simulink model "ThreePhase_FullControlRectifier"  (R2020a)
settings: Solver=VariableStepAuto  StartTime=0.0  StopTime=0.0335  RelTol=1e-3
libraries: powerlib x15
settings Model: Creator=Naeem Mohammad  LastModifiedBy=Naeem Mohammad

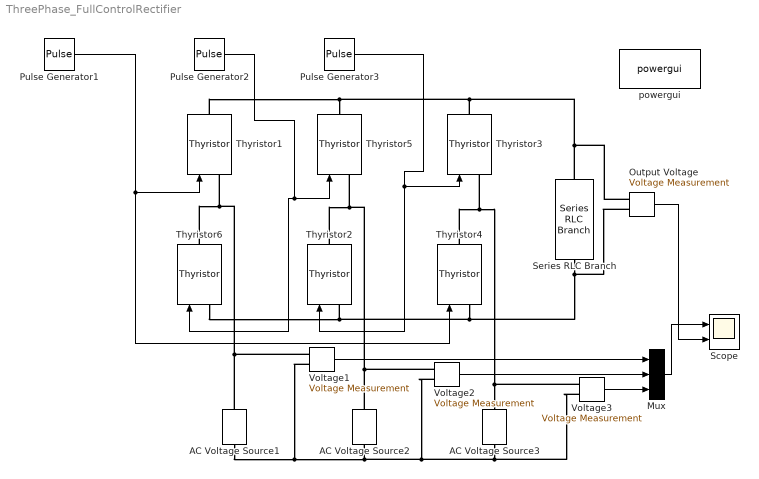
== system ThreePhase_FullControlRectifier ==
  AC Voltage Source1 : powerlib/Electrical Sources/AC Voltage Source  Amplitude=220  Phase=0  Frequency=60  SampleTime=0  Measurements=None  BusType=swing  Pref=10e3  Qref=0  Qmin=-inf  Qmax=+inf
  AC Voltage Source2 : powerlib/Electrical Sources/AC Voltage Source  Amplitude=220  Phase=120  Frequency=60  SampleTime=0  Measurements=None  BusType=swing  Pref=10e3  Qref=0  Qmin=-inf  Qmax=+inf
  AC Voltage Source3 : powerlib/Electrical Sources/AC Voltage Source  Amplitude=220  Phase=240  Frequency=60  SampleTime=0  Measurements=None  BusType=swing  Pref=10e3  Qref=0  Qmin=-inf  Qmax=+inf
  Mux : Mux  Inputs=3
  Output Voltage : powerlib/Measurements/Voltage Measurement  PhasorSimulation=off  OutputType=Complex  PSBequivalent=0
  Pulse Generator1 : DiscretePulseGenerator  PulseType=Time based  Period=1/60  PulseWidth=5  PhaseDelay=45*(1/60)*(1/360)
  Pulse Generator2 : DiscretePulseGenerator  PulseType=Time based  Period=1/60  PulseWidth=5  PhaseDelay=165*(1/60)*(1/360)
  Pulse Generator3 : DiscretePulseGenerator  PulseType=Time based  Period=1/60  PulseWidth=5  PhaseDelay=285*(1/60)*(1/360)
  Scope : Scope  NumInputPorts=2
  Series RLC Branch : powerlib/Elements/Series RLC Branch  LConnTagsString=__new0  RConnTagsString=__new0  BranchType=R  Resistance=1  Inductance=650e-3  SetiL0=off  InitialCurrent=0  Capacitance=1e-6  Setx0=off  InitialVoltage=0  Measurements=None
  Thyristor{1..6} (6 alike) : powerlib/Power Electronics/Thyristor  Ron=0.001  Lon=0  Vf=0.8  IC=0  Rs=500  Cs=250e-9  Measurements=off
  Voltage1 : powerlib/Measurements/Voltage Measurement  PhasorSimulation=off  OutputType=Complex  PSBequivalent=0
  Voltage2 : powerlib/Measurements/Voltage Measurement  PhasorSimulation=off  OutputType=Complex  PSBequivalent=0
  Voltage3 : powerlib/Measurements/Voltage Measurement  PhasorSimulation=off  OutputType=Complex  PSBequivalent=0
  powergui : powerlib/powergui  Priority=1  SimulationMode=Continuous  SampleTime=50e-6  frequency=60  Iterations=50  frequencyindice=60  Pbase=100e6  ErrMax=1e-4  UnitsV=kV  UnitsW=MW  buscounter=0  FunctionMessages=off  echomessages=off  EnableUseOfTLC=off  CurrentSourceSwitches=off  DisableSnubberDevices=off  DisableRonSwitches=off  DisableVfSwitches=off  DisplayEquations=off  AutomaticDiscreteSolvers=off  SolverType=Tustin/Backward Euler (TBE)  Interpol=off  ExternalGateDelay=off  methode=off  Ts=100  x0status=blocks  SPID=on  SwTol=0  HookPort=off  NonlinearTolerance=1e-4  nMaxIteration=100  ContinueOnMaxIteration=off  RestoreLinks=warning  ResistiveCurrentMeasurement=off  Frange=[0:2:500]  Ylog=off  Xlog=on  ShowGrid=off  save=off  variable=ZData  structure=0  ZoomFFT=off  StartTime=0.0  cycles=1  DisplayStyle=1  fundamental=60  FreqAxis=off  MaxFrequency=1000  frequencyindicesteady=1  RmsSteady=1  display=off
  wires:
  Pulse Generator1/1 -> Thyristor1/1, Thyristor4/1
  Pulse Generator2/1 -> Thyristor6/1, Thyristor5/1
  Pulse Generator3/1 -> Thyristor3/1, Thyristor2/1
  Voltage1/1 -> Mux/1
  Voltage2/1 -> Mux/2
  Voltage3/1 -> Mux/3
  Mux/1 -> Scope/1
  Output Voltage/1 -> Scope/2
  connections:
  Thyristor6/RConn1 -- AC Voltage Source1/RConn1 -- Voltage1/LConn1 -- Thyristor1/LConn1
  Thyristor2/RConn1 -- Voltage2/LConn1 -- AC Voltage Source2/RConn1 -- Thyristor5/LConn1
  Thyristor6/LConn1 -- Output Voltage/LConn2 -- Series RLC Branch/RConn1 -- Thyristor4/LConn1 -- Thyristor2/LConn1
  Thyristor1/RConn1 -- Series RLC Branch/LConn1 -- Output Voltage/LConn1 -- Thyristor3/RConn1 -- Thyristor5/RConn1
  Thyristor4/RConn1 -- Voltage3/LConn1 -- AC Voltage Source3/RConn1 -- Thyristor3/LConn1
  AC Voltage Source1/LConn1 -- Voltage3/LConn2 -- AC Voltage Source3/LConn1 -- Voltage2/LConn2 -- AC Voltage Source2/LConn1 -- Voltage1/LConn2
